simulink model "W3_Problem_2"  (R2020a)
settings: Solver=VariableStepAuto  StartTime=0.0  StopTime=10.0  RelTol=1e-3
undefined symbols (not defined in the file): DiscIntNeverNeededParam
libraries: simulink x1
settings Model: Creator=user  LastModifiedBy=user

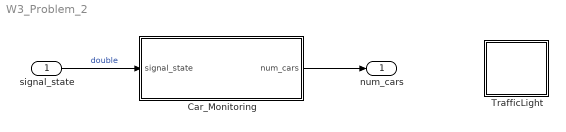
== system W3_Problem_2 ==
  signal_state : Inport
  Car_Monitoring : Subsystem
  TrafficLight : Stateflow chart  TreatAsAtomicUnit=on
  num_cars : Outport  VectorParamsAs1DForOutWhenUnconnected=off
  wires:
  signal_state/1 -> Car_Monitoring/1(signal_state)  "double"
  Car_Monitoring/1(num_cars) -> num_cars/1

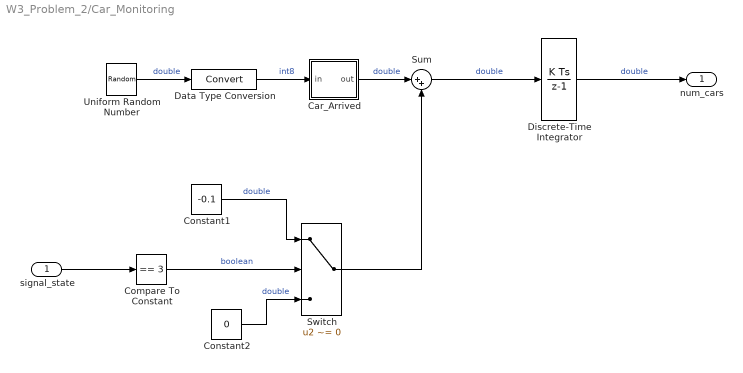
== system W3_Problem_2/Car_Monitoring ==
  signal_state : Inport
  Car_Arrived : Stateflow chart  TreatAsAtomicUnit=on
  Compare To Constant : simulink/Logic and Bit Operations/Compare To Constant  relop===  const=3  OutDataTypeStr=boolean  ZeroCross=off
  Constant1 : Constant  Value=-0.1
  Constant2 : Constant  Value=0
  Data Type Conversion : DataTypeConversion
  Discrete-Time Integrator : DiscreteIntegrator  SampleTime=-1  LimitOutput=on  LowerSaturationLimit=0  ICPrevOutput=DiscIntNeverNeededParam  ICPrevScaledInput=DiscIntNeverNeededParam
  Sum : Sum  Inputs=|++
  Switch : Switch  Criteria=u2 ~= 0
  Uniform Random Number : UniformRandomNumber  Minimum=0  Maximum=100  Seed=177836  SampleTime=0
  num_cars : Outport  VectorParamsAs1DForOutWhenUnconnected=off
  wires:
  Switch/1 -> Sum/2
  Car_Arrived/1(out) -> Sum/1  "double"
  Data Type Conversion/1 -> Car_Arrived/1(in)  "int8"
  Compare To Constant/1 -> Switch/2  "boolean"
  Constant2/1 -> Switch/3  "double"
  signal_state/1 -> Compare To Constant/1
  Uniform Random Number/1 -> Data Type Conversion/1  "double"
  Constant1/1 -> Switch/1  "double"
  Discrete-Time Integrator/1 -> num_cars/1  "double"
  Sum/1 -> Discrete-Time Integrator/1  "double"

== stateflow chart W3_Problem_2/Car_Monitoring/Car_Arrived ==
  (default) -> (junction 1) : {out = in > 98;}
  data: in input; out output

== stateflow chart W3_Problem_2/TrafficLight ==
  settings: stateMachineType=MOORE_MACHINE
  state Stop
    y1 = RED;
    y2 = GREEN;
  state StopForTrafic
    y1 = RED;
    y2 = GREEN;
  state StopToGo
    y1 = RED;
    y2 = YELLOW;
  state GoToStop
    y1 = YELLOW;
    y2 = RED;
  state Go
    y1 = GREEN;
    y2 = RED;
  (default) -> Stop
  Stop -> StopForTrafic : after(20,tick)
  StopForTrafic -> StopToGo : [sens]
  GoToStop -> Stop : after(3,tick)
  StopToGo -> Go : after(3,tick)
  Go -> GoToStop : after(10,tick)
